simulink model "FlyBackConv"  (R2021b)
settings: Solver=ode4  StartTime=0.0  StopTime=3e-4  FixedStep=1e-9  RelTol=1e-3
values from neighbouring files (symbols this model uses):
  C = D/fs*(Vc-Vbat)/Rout/delVc    (= 1.03597563342e-05)    [Script.m]
  fs = 250e3    (= 250000)    [Script.m]
  Gcinf = (abs(evalfr(Tuiind,1i*2*pi*fc)))/sqrt(1+(wLv/2/pi/fc)^2)/abs(evalfr(Gfilter,1i*2*pi*fc))    [Script.m]
  Lm = Vc*Dp/delIlm/fs    (= 0.000738946619669)    [Script.m]
  Rin = 100e-3    (= 0.1)    [Script.m]
  Rout = Rin    (= 0.1)    [Script.m]
  Rsense = 5/0.2    (= 25)    [Script.m]
  Vbat = 3.7    [Script.m]
  Vin = 3.7    [Script.m]
  Vm = 5    [Script.m]
  wLv = 2*pi*fc*tan(75*pi/180)    [Script.m]
  wpfilter = 2*pi*30e3    (= 188495.559215)    [Script.m]
libraries: spsCurrentMeasurementLib x4, spsSeriesRLCBranchLib x4, spsVoltageMeasurementLib x4, spsDCVoltageSourceLib x2, spsMosfetLib x2, spsLinearTransformerLib x1, simulink x1, spspowerguiLib x1
settings Model: SimulationMode=rapid-accelerator  Creator=Aditya Bhalotia  LastModifiedBy=ee3210698
settings DebuggingCC: UnconnectedInputMsg=none  UnconnectedOutputMsg=none  UnconnectedLineMsg=none
settings RTWCC: DLArmComputeVersion=20.02.1

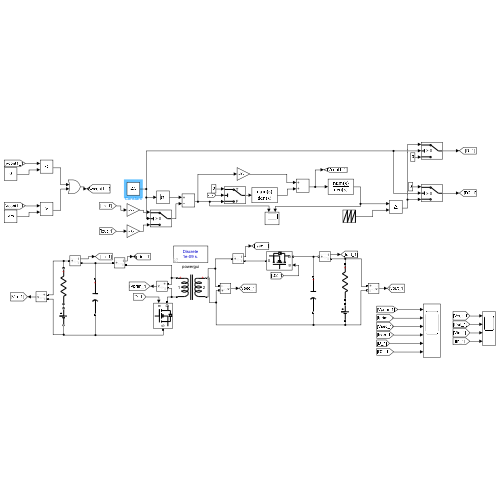
[thumbnail: Simulink's stored preview of the top-level diagram]
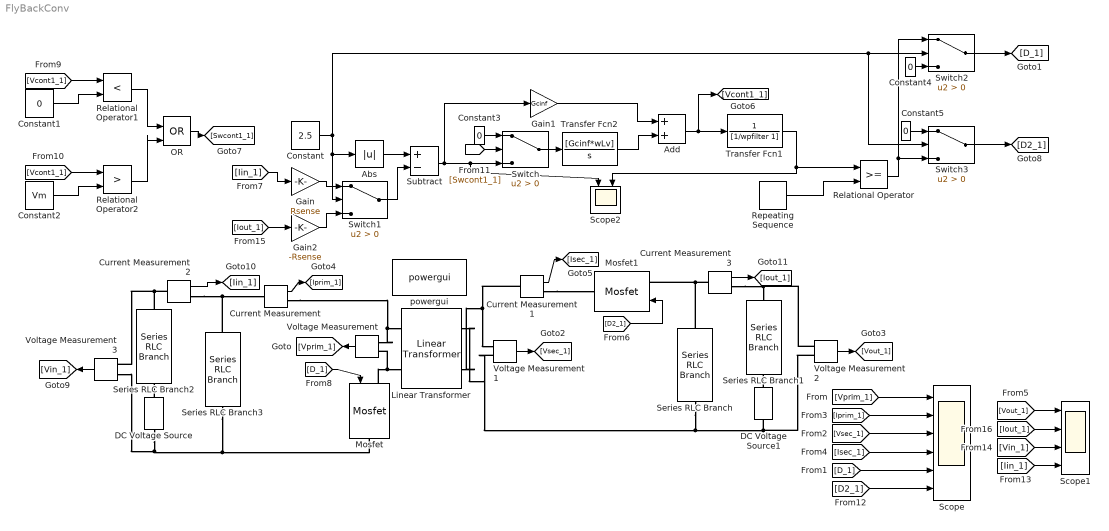
== system FlyBackConv ==
  Abs : Abs
  Add : Sum
  Constant : Constant  Value=2.5
  Constant{1,3..5} (4 alike) : Constant  Value=0
  Constant2 : Constant  Value=Vm
  Current Measurement{,1..3} (4 alike) : spsCurrentMeasurementLib/Current Measurement  PhasorSimulation=off  OutputType=Complex  PSBequivalent=0
  DC Voltage Source : spsDCVoltageSourceLib/DC Voltage Source  Amplitude=Vin  Measurements=None
  DC Voltage Source1 : spsDCVoltageSourceLib/DC Voltage Source  Amplitude=Vbat  Measurements=None
  Gain : Gain  Gain=Rsense
  Gain1 : Gain  Gain=Gcinf
  Gain2 : Gain  Gain=-Rsense
  Linear Transformer : spsLinearTransformerLib/Linear Transformer  UNITS=SI  NominalPower=[ 200 250e3 ]  winding1=[10 0.1 0]  winding2=[10 0 0]  ThreeWindings=off  winding3=[3.15e+05 0.7938 0.084225]  RmLm=[inf Lm]  Measurements=None  DataType=on
  Mosfet : spsMosfetLib/Mosfet  Ron=0.001  Lon=0  Rd=0.001  Vfd=0  IC=0  Rs=10e9  Cs=inf  Measurements=off
  Mosfet1 : spsMosfetLib/Mosfet  Ron=0.001  Lon=0  Rd=0.001  Vfd=0  IC=0  Rs=10e9  Cs=inf  Measurements=off
  OR : Logic  Operator=OR  IconShape=distinctive  AllPortsSameDT=off  OutDataTypeStr=boolean
  Relational Operator : RelationalOperator  OutDataTypeStr=boolean  RndMeth=Simplest
  Relational Operator1 : RelationalOperator  Operator=<  OutDataTypeStr=boolean  RndMeth=Simplest
  Relational Operator2 : RelationalOperator  Operator=>  OutDataTypeStr=boolean  RndMeth=Simplest
  Repeating Sequence : simulink/Sources/Repeating Sequence  rep_seq_t=[0 1/fs]  rep_seq_y=[0 Vm]
  Scope : Scope  NumInputPorts=6
  Scope1 : Scope  NumInputPorts=4
  Scope2 : Scope  NumInputPorts=2
  Series RLC Branch : spsSeriesRLCBranchLib/Series RLC Branch  LConnTagsString=__new0  RConnTagsString=__new0  BranchType=C  Resistance=1  Inductance=1e-3  SetiL0=off  InitialCurrent=0  Capacitance=C  Setx0=off  InitialVoltage=0  Measurements=None
  Series RLC Branch1 : spsSeriesRLCBranchLib/Series RLC Branch  LConnTagsString=__new0  RConnTagsString=__new0  BranchType=R  Resistance=Rout  Inductance=1e-3  SetiL0=off  InitialCurrent=0  Capacitance=1e-6  Setx0=off  InitialVoltage=0  Measurements=None
  Series RLC Branch2 : spsSeriesRLCBranchLib/Series RLC Branch  LConnTagsString=__new0  RConnTagsString=__new0  BranchType=R  Resistance=Rin  Inductance=1e-3  SetiL0=off  InitialCurrent=0  Capacitance=1e-6  Setx0=off  InitialVoltage=0  Measurements=None
  Series RLC Branch3 : spsSeriesRLCBranchLib/Series RLC Branch  LConnTagsString=__new0  RConnTagsString=__new0  BranchType=C  Resistance=1  Inductance=1e-3  SetiL0=off  InitialCurrent=0  Capacitance=C  Setx0=off  InitialVoltage=0  Measurements=None
  Subtract : Sum  Inputs=+-
  Switch{,1..3} (4 alike) : Switch  Criteria=u2 > Threshold
  Transfer Fcn1 : TransferFcn  Denominator=[1/wpfilter 1]
  Transfer Fcn2 : TransferFcn  Numerator=[Gcinf*wLv]  Denominator=[1 0]
  Voltage Measurement{,1..3} (4 alike) : spsVoltageMeasurementLib/Voltage Measurement  PhasorSimulation=off  OutputType=Complex  PSBequivalent=0
  powergui : spspowerguiLib/powergui  Priority=1  SimulationMode=Discrete  SampleTime=1e-9  frequency=60  Iterations=50  frequencyindice=0  Pbase=100e6  ErrMax=1e-4  UnitsV=kV  UnitsW=MW  buscounter=0  FunctionMessages=off  echomessages=off  EnableUseOfTLC=off  CurrentSourceSwitches=off  DisableSnubberDevices=off  DisableRonSwitches=off  DisableVfSwitches=off  DisplayEquations=off  AutomaticDiscreteSolvers=off  SolverType=Tustin/Backward Euler (TBE)  Interpol=off  ExternalGateDelay=off  methode=off  Ts=100  x0status=blocks  SPID=on  SwTol=0  HookPort=off  NonlinearTolerance=1e-4  nMaxIteration=100  ContinueOnMaxIteration=off  RestoreLinks=warning  ResistiveCurrentMeasurement=off  Frange=[0:2:500]  Ylog=off  Xlog=on  ShowGrid=off  save=off  variable=ZData  structure=0  ZoomFFT=off  StartTime=0.0  cycles=1  DisplayStyle=1  fundamental=60  FreqAxis=off  MaxFrequency=1000  frequencyindicesteady=1  RmsSteady=1  display=off
  wires:
  Voltage Measurement/1 -> [Vprim_1]
  [Vprim_1] -> Scope/1
  [D_1] -> Scope/5
  Voltage Measurement1/1 -> [Vsec_1]
  [Vsec_1] -> Scope/3
  Current Measurement/1 -> [Iprim_1]
  [Iprim_1] -> Scope/2
  [Isec_1] -> Scope/4
  Current Measurement1/1 -> [Isec_1]
  [Vout_1] -> Scope1/1
  Voltage Measurement2/1 -> [Vout_1]
  [Iin_1] -> Gain/1
  Constant/1 -> Switch1/2, Abs/1, Switch3/2, Switch2/2
  Subtract/1 -> Switch/3, Scope2/1, Gain1/1
  Transfer Fcn1/1 -> Scope2/2, Relational Operator/1
  Repeating Sequence/1 -> Relational Operator/2
  [D_1] -> Mosfet/1
  Gain1/1 -> Add/1
  Switch/1 -> Transfer Fcn2/1
  Add/1 -> Transfer Fcn1/1, [Vcont1_1]
  [Vcont1_1] -> Relational Operator1/1
  Constant1/1 -> Relational Operator1/2
  Constant2/1 -> Relational Operator2/2
  [Vcont1_1] -> Relational Operator2/1
  Relational Operator1/1 -> OR/1
  Relational Operator2/1 -> OR/2
  OR/1 -> [Swcont1_1]
  [Swcont1_1] -> Switch/2
  Constant3/1 -> Switch/1
  Transfer Fcn2/1 -> Add/2
  [Iout_1] -> Gain2/1
  Gain/1 -> Switch1/1
  Gain2/1 -> Switch1/3
  Switch1/1 -> Subtract/2
  Relational Operator/1 -> Switch2/1, Switch3/3
  Switch2/1 -> [D_1]
  Constant4/1 -> Switch2/3
  Constant5/1 -> Switch3/1
  Switch3/1 -> [D2_1]
  [D2_1] -> Mosfet1/1
  Abs/1 -> Subtract/1
  [D2_1] -> Scope/6
  Voltage Measurement3/1 -> [Vin_1]
  [Vin_1] -> Scope1/3
  Current Measurement2/1 -> [Iin_1]
  Current Measurement3/1 -> [Iout_1]
  [Iin_1] -> Scope1/4
  [Iout_1] -> Scope1/2
  connections:
  DC Voltage Source/LConn1 -- Mosfet/RConn1 -- Series RLC Branch3/RConn1 -- Voltage Measurement3/LConn2
  Mosfet/LConn1 -- Voltage Measurement/LConn2 -- Linear Transformer/LConn2
  Voltage Measurement/LConn1 -- Current Measurement/RConn1 -- Linear Transformer/LConn1
  Series RLC Branch/LConn1 -- Mosfet1/LConn1 -- Current Measurement3/LConn1
  Series RLC Branch/RConn1 -- Linear Transformer/RConn1 -- Voltage Measurement1/LConn1 -- DC Voltage Source1/LConn1 -- Voltage Measurement2/LConn2
  DC Voltage Source/RConn1 -- Series RLC Branch2/RConn1
  Current Measurement1/LConn1 -- Voltage Measurement1/LConn2 -- Linear Transformer/RConn2
  Current Measurement1/RConn1 -- Mosfet1/RConn1
  DC Voltage Source1/RConn1 -- Series RLC Branch1/RConn1
  Series RLC Branch3/LConn1 -- Current Measurement/LConn1 -- Current Measurement2/RConn1
  Current Measurement2/LConn1 -- Series RLC Branch2/LConn1 -- Voltage Measurement3/LConn1
  Voltage Measurement2/LConn1 -- Current Measurement3/RConn1 -- Series RLC Branch1/LConn1
